simulink model "tanksimulation"  (R2023b)
settings: Solver=VariableStepAuto  StartTime=0.0  StopTime=20  RelTol=1e-3
values from neighbouring files (symbols this model uses):
  A = [-1/(R1*C1) 1/(R1*C1) ... (first row only)    [coupledtank.m]
  B = [1/C1 0 ... (first row only)    [coupledtank.m]
  C = eye(2)    [coupledtank.m]
  K = lqr(A_bar,B_bar,Q,R)    [coupledtank.m]
settings Model: LastModifiedBy=91798

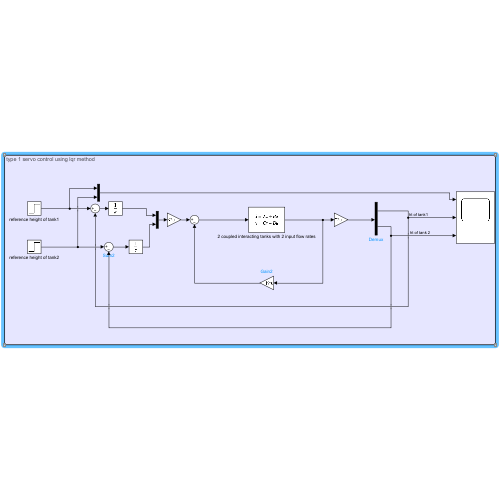
[thumbnail: Simulink's stored preview of the top-level diagram]
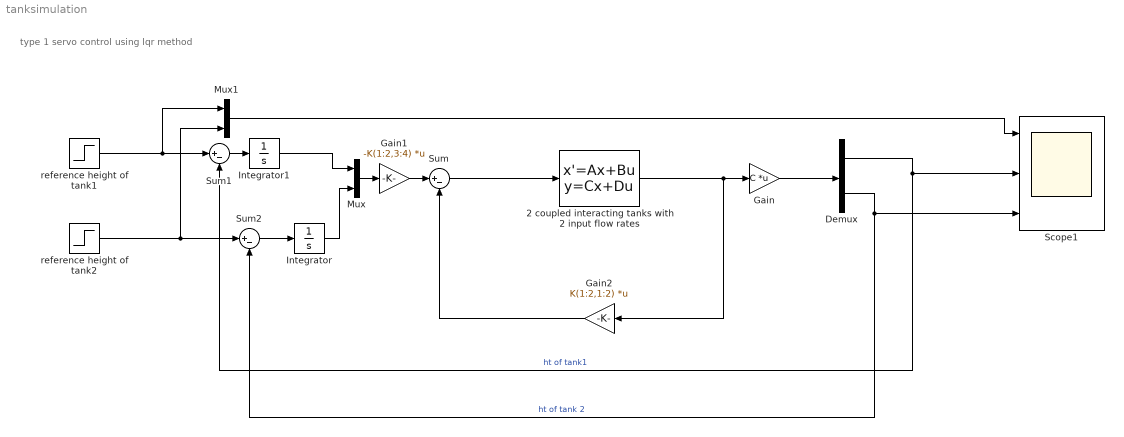
== system tanksimulation ==
  note: type 1 servo control using lqr method
  2 coupled interacting tanks with 2 input flow rates : StateSpace  A=A  B=B  C=eye(2)  D=zeros(2)  InitialCondition=0
  Demux : Demux  Outputs=2
  Gain : Gain  Gain=C  Multiplication=Matrix(K*u)
  Gain1 : Gain  Gain=-K(1:2,3:4)  Multiplication=Matrix(K*u)
  Gain2 : Gain  Gain=K(1:2,1:2)  Multiplication=Matrix(K*u)
  Integrator : Integrator
  Integrator1 : Integrator
  Mux : Mux  Inputs=2
  Mux1 : Mux  Inputs=2
  Scope1 : Scope  NumInputPorts=3
  Sum : Sum  Inputs=|+-
  Sum1 : Sum  Inputs=|+-
  Sum2 : Sum  Inputs=|+-
  reference height of tank1 : Step  After=2  SampleTime=0
  reference height of tank2 : Step  SampleTime=0
  wires:
  2 coupled interacting tanks with 2 input flow rates/1 -> Gain2/1, Gain/1
  Gain/1 -> Demux/1
  Demux/1 -> Sum1/2, Scope1/2  "ht of tank1"
  Demux/2 -> Sum2/2, Scope1/3  "ht of tank 2"
  Integrator1/1 -> Mux/1
  Integrator/1 -> Mux/2
  Sum/1 -> 2 coupled interacting tanks with 2 input flow rates/1
  Mux/1 -> Gain1/1
  Gain2/1 -> Sum/2
  Gain1/1 -> Sum/1
  reference height of tank2/1 -> Mux1/2, Sum2/1
  Sum1/1 -> Integrator1/1
  Sum2/1 -> Integrator/1
  reference height of tank1/1 -> Mux1/1, Sum1/1
  Mux1/1 -> Scope1/1
